simulink model "prelab1simulink"  (R2019b)
settings: Solver=ode45  StartTime=0.0  StopTime=10.0  MaxStep=1e-3  RelTol=1e-3
settings Model: Creator=wesle  LastModifiedBy=wesle

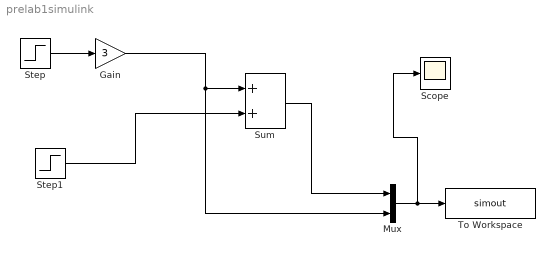
== system prelab1simulink ==
  Gain : Gain  Gain=3
  Mux : Mux  Inputs=2
  Scope : Scope
  Step : Step  After=3  SampleTime=0
  Step1 : Step  Time=4  After=4  SampleTime=0
  Sum : Sum
  To Workspace : ToWorkspace  VariableName=simout  SampleTime=-1
  wires:
  Step/1 -> Gain/1
  Step1/1 -> Sum/2
  Sum/1 -> Mux/1
  Gain/1 -> Mux/2, Sum/1
  Mux/1 -> Scope/1, To Workspace/1
